simulink model "Lab7_pkt3"  (R2017a)
settings: Solver=VariableStepAuto  StartTime=0.0  StopTime=10.0  RelTol=1e-3
values from neighbouring files (symbols this model uses):
  t0 = (k - b)/a    [Lab4.m]    (also in Lab7.m = 71.2)
libraries: cstblocks x4
settings Model: Creator=ishiguro  LastModifiedBy=ishiguro

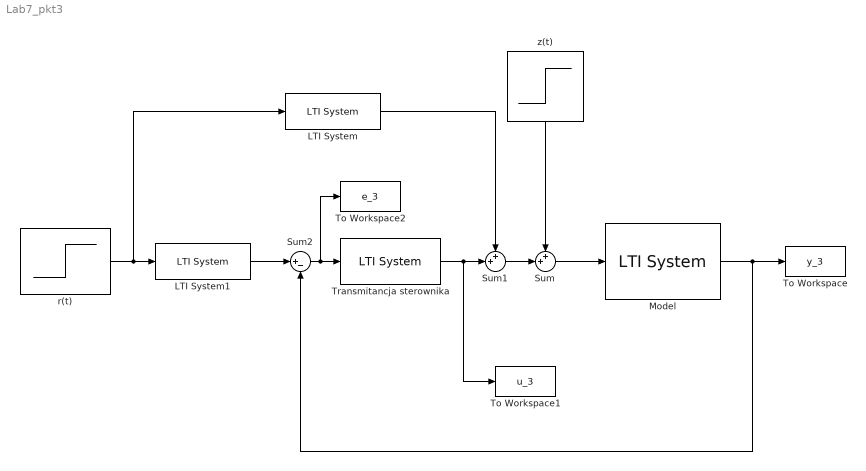
== system Lab7_pkt3 ==
  LTI System : cstblocks/LTI System  sys=Kff  IC=[]
  LTI System1 : cstblocks/LTI System  sys=Gm  IC=[]
  Model : cstblocks/LTI System  sys=K  IC=[]
  Sum : Sum  Inputs=++|
  Sum1 : Sum  Inputs=++|
  Sum2 : Sum  Inputs=|+-
  To Workspace : ToWorkspace  VariableName=y_3  SampleTime=-1
  To Workspace1 : ToWorkspace  VariableName=u_3  SampleTime=-1
  To Workspace2 : ToWorkspace  VariableName=e_3  SampleTime=-1
  Transmitancja sterownika : cstblocks/LTI System  sys=Kr3  IC=[]
  r(t) : Step  Time=0  SampleTime=0
  z(t) : Step  Time=t0  SampleTime=0
  wires:
  Transmitancja sterownika/1 -> Sum1/2, To Workspace1/1
  Model/1 -> Sum2/2, To Workspace/1
  Sum/1 -> Model/1
  r(t)/1 -> LTI System1/1, LTI System/1
  LTI System/1 -> Sum1/1
  z(t)/1 -> Sum/1
  Sum1/1 -> Sum/2
  Sum2/1 -> To Workspace2/1, Transmitancja sterownika/1
  LTI System1/1 -> Sum2/1
